simulink model "DC_MotorEquation_Encoder"  (R2024b)
settings: Solver=VariableStepAuto  StartTime=0.0  StopTime=10  FixedStep=0.0001  RelTol=1e-3
undefined symbols (not defined in the file): b, J, Km, L, PulseNumber, R, RadiantsPerCount, RadToRpm, Tau_I, TSample
settings Model: Creator=Davide  LastModifiedBy=Utente
settings DataIOCC: ReturnWorkspaceOutputs=off
settings OptimizationCC: ReuseModelBlockBuffer=off
settings RTWCC: GPUComputeCapability=3.5

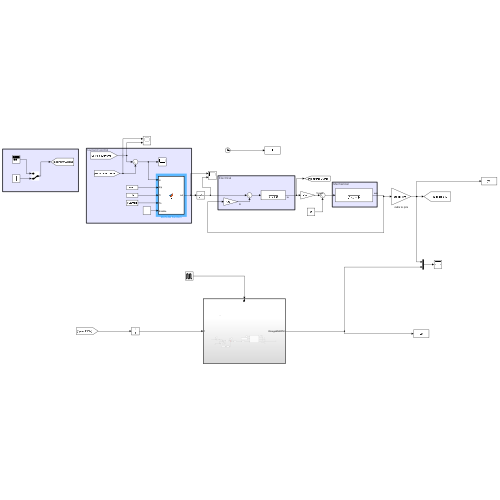
[thumbnail: Simulink's stored preview of the top-level diagram]
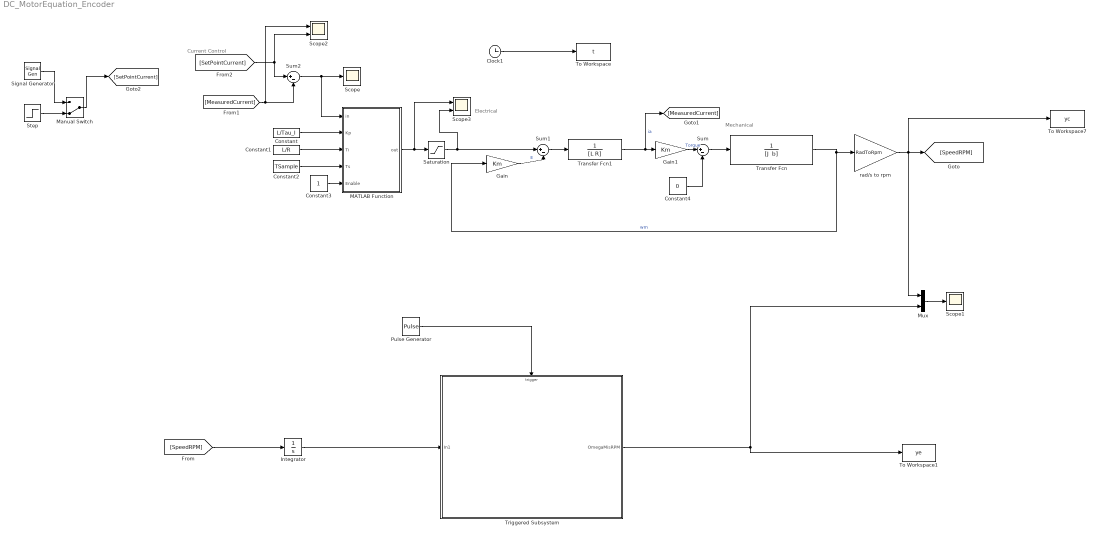
== system DC_MotorEquation_Encoder ==
  note: Current Control
  note: Electrical
  note: Mechanical
  Clock1 : Clock
  Constant : Constant  Value=L/Tau_I
  Constant1 : Constant  Value=L/R
  Constant2 : Constant  Value=TSample
  Constant3 : Constant
  Constant4 : Constant  Value=0
  Gain : Gain  Gain=Km
  Gain1 : Gain  Gain=Km
  Integrator : Integrator
  MATLAB Function : MATLAB Function  TreatAsAtomicUnit=on  SystemSampleTime=TSample
  Manual Switch : ManualSwitch  CurrentSetting=0
  Mux : Mux  Inputs=2
  Pulse Generator : DiscretePulseGenerator  PulseType=Time based  Period=TSample  PulseWidth=50
  Saturation : Saturate  UpperLimit=+24  LowerLimit=-24
  Scope : Scope
  Scope1 : Scope
  Scope2 : Scope  NumInputPorts=2
  Scope3 : Scope  NumInputPorts=2
  Signal Generator : SignalGenerator  WaveForm=square  Frequency=0.05
  Step : Step  Time=0  After=0.5  SampleTime=0
  Sum : Sum  Inputs=|+-
  Sum1 : Sum  Inputs=|+-
  Sum2 : Sum  Inputs=|+-
  To Workspace : ToWorkspace  VariableName=t  SampleTime=-1
  To Workspace1 : ToWorkspace  VariableName=ye  SampleTime=-1
  To Workspace7 : ToWorkspace  VariableName=yc  SampleTime=-1
  Transfer Fcn : TransferFcn  Denominator="[J  b]"
  Transfer Fcn1 : TransferFcn  Denominator=[L R]
  Triggered Subsystem : Subsystem  TreatAsAtomicUnit=on
  rad/s to rpm : Gain  Gain=RadToRpm  SaturateOnIntegerOverflow=on  OutDataTypeStr=Inherit: Same as input  ParamDataTypeStr=Inherit: Same as input
  wires:
  Signal Generator/1 -> Manual Switch/1
  Gain1/1 -> Sum/1  "Torque"
  Transfer Fcn/1 -> Gain/1, rad/s to rpm/1  "wm"
  Transfer Fcn1/1 -> Gain1/1, [MeasuredCurrent]  "ia"
  Sum1/1 -> Transfer Fcn1/1
  Pulse Generator/1 -> Triggered Subsystem/Trigger
  Integrator/1 -> Triggered Subsystem/1(In1)
  [SpeedRPM] -> Integrator/1
  Step/1 -> Manual Switch/2
  Manual Switch/1 -> [SetPointCurrent]
  rad/s to rpm/1 -> To Workspace7/1, [SpeedRPM], Mux/1
  Triggered Subsystem/1(OmegaMisRPM) -> To Workspace1/1, Mux/2
  Mux/1 -> Scope1/1
  Clock1/1 -> To Workspace/1
  MATLAB Function/1(out) -> Scope3/1, Saturation/1
  Sum2/1 -> MATLAB Function/1(in), Scope/1
  Constant/1 -> MATLAB Function/2(Kp)
  Constant1/1 -> MATLAB Function/3(Ti)
  Constant2/1 -> MATLAB Function/4(Ts)
  Constant3/1 -> MATLAB Function/5(Enable)
  Saturation/1 -> Sum1/1, Scope3/2
  Sum/1 -> Transfer Fcn/1
  Constant4/1 -> Sum/2
  [MeasuredCurrent] -> Sum2/2, Scope2/1
  [SetPointCurrent] -> Scope2/2, Sum2/1
  Gain/1 -> Sum1/2  "E"

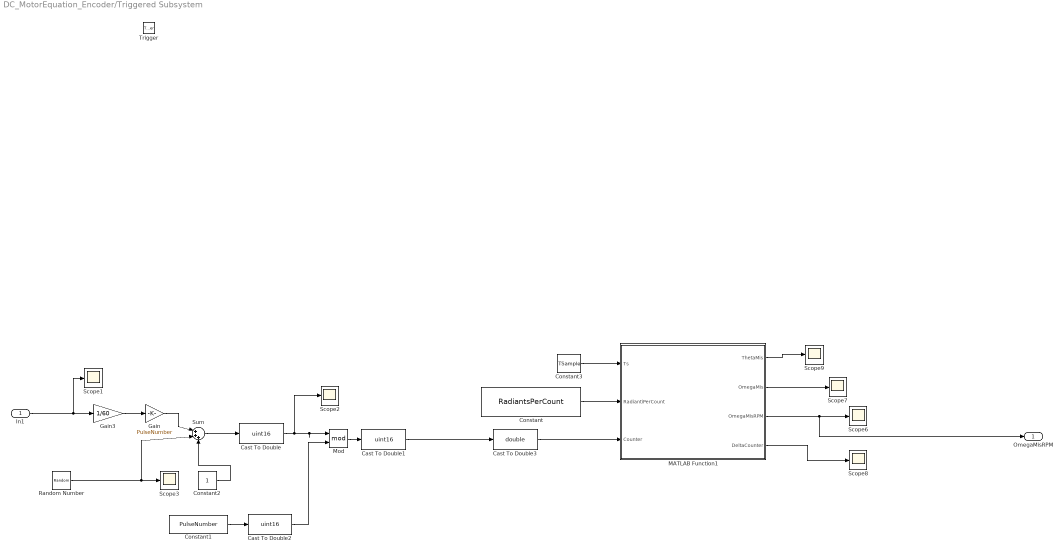
== system DC_MotorEquation_Encoder/Triggered Subsystem ==
  In1 : Inport
  Trigger : TriggerPort  VariantControl=(inherit)
  Cast To Double : DataTypeConversion  OutDataTypeStr=uint16  SaturateOnIntegerOverflow=off  RndMeth=Floor
  Cast To Double1 : DataTypeConversion  OutDataTypeStr=uint16  SaturateOnIntegerOverflow=off  RndMeth=Floor
  Cast To Double2 : DataTypeConversion  OutDataTypeStr=uint16  SaturateOnIntegerOverflow=off  RndMeth=Floor
  Cast To Double3 : DataTypeConversion  OutDataTypeStr=double  SaturateOnIntegerOverflow=off  RndMeth=Floor
  Constant : Constant  Value=RadiantsPerCount
  Constant1 : Constant  Value=PulseNumber
  Constant2 : Constant
  Constant3 : Constant  Value=TSample
  Gain : Gain  Gain=PulseNumber
  Gain3 : Gain  Gain=1/60
  MATLAB Function1 : MATLAB Function  TreatAsAtomicUnit=on
  Mod : Math  Operator=mod
  Random Number : RandomNumber  Variance=0.3
  Scope{1..3,6..9} (7 alike) : Scope
  Sum : Sum  Inputs=|+++
  OmegaMisRPM : Outport
  wires:
  Cast To Double2/1 -> Mod/2
  Cast To Double/1 -> Scope2/1, Mod/1
  Constant1/1 -> Cast To Double2/1
  Mod/1 -> Cast To Double1/1
  Cast To Double1/1 -> Cast To Double3/1
  Gain/1 -> Sum/1
  Constant/1 -> MATLAB Function1/2(RadiantiPerCount)
  Constant3/1 -> MATLAB Function1/1(Ts)
  MATLAB Function1/3(OmegaMisRPM) -> OmegaMisRPM/1, Scope6/1
  Cast To Double3/1 -> MATLAB Function1/3(Counter)
  MATLAB Function1/1(ThetaMis) -> Scope9/1
  MATLAB Function1/2(OmegaMis) -> Scope7/1
  MATLAB Function1/4(DeltaCounter) -> Scope8/1
  Gain3/1 -> Gain/1
  In1/1 -> Scope1/1, Gain3/1
  Sum/1 -> Cast To Double/1
  Random Number/1 -> Scope3/1, Sum/2
  Constant2/1 -> Sum/3

== matlab function DC_MotorEquation_Encoder/MATLAB Function ==
  data: in input; out output; Kp input; Ti input; Ts input; Enable input
function out = PI( in ,Kp , Ti , Ts , Enable)
persistent in_prev out_prev
% Initial Value
if isempty( out_prev )
out_prev = 0;
end
if isempty( in_prev )
in_prev = 0;
end
% G(s)=(Kp/Ti)*((1+Ti*s)/s) (Tustin)
% We run control only if motor is running
if (Enable == 1)
%I Calculate the output
 out = Kp*Ts/(2*Ti)*(in+in_prev) + Kp*(in-in_prev) + out_prev;
else
out = 0;
in = 0;
end
out_prev = out;
in_prev = in;
end

== matlab function DC_MotorEquation_Encoder/Triggered Subsystem/MATLAB Function1 ==
  data: Ts input; ThetaMis output; RadiantiPerCount input; Counter input; OmegaMis output; OmegaMisRPM output; DeltaCounter output
function [ThetaMis, OmegaMis, OmegaMisRPM, DeltaCounter] = CounterToThetaOmega(Ts, RadiantiPerCount, Counter)

% Inizializzazione dei valori iniziali 
persistent CounterPrec  
if isempty( CounterPrec )
    CounterPrec = 0;
end 

    DeltaCounter=Counter-CounterPrec;
    
    if (DeltaCounter>double(0x1000))
        DeltaCounter=DeltaCounter-double(0x2000);
    end
    
    if (DeltaCounter<-double(0x1000))
        DeltaCounter=DeltaCounter+double(0x2000);
    end
        
    % conversione conteggio in radianti
    ThetaMis = Counter * RadiantiPerCount;
    
    DeltaThetaMis = DeltaCounter*RadiantiPerCount;
   
    OmegaMis = DeltaThetaMis/Ts;
    OmegaMisRPM=OmegaMis*60/(2*pi);
 
    CounterPrec= Counter;
end
